simulink model "HSM_4p6U10_Motion_v01_06022022_NEW_ECC_2019a"  (R2019a)
settings: Solver=ode1  StartTime=0.0  StopTime=Inf  FixedStep=Ts  RelTol=1e-3  EnableMultiTasking=on
PostLoadFcn:
  | , if any(exist('dsrtsu_mdlpostloadfcn', 'file') == [2, 3, 6]), try dsrtsu_mdlpostloadfcn('Execute', bdroot); catch fprintf('Error in PostLoadFcn (dsrtsu_mdlpostloadfcn) for model "%s":\n %s\n', bdroot, lasterr); end, end,
values from neighbouring files (symbols this model uses):
  CDP = -1    [Parameters_4p6U10.m]
  CUP = 1    [Parameters_4p6U10.m]
  HDP = 1    [Parameters_4p6U10.m]
  HUP = -1    [Parameters_4p6U10.m]
  K1m = 1.7E-4    (= 0.00017)    [Parameters_4p6U10.m]
  K2m = 7.0E-4    (= 0.0007)    [Parameters_4p6U10.m]
  Ts = 0.0002    [Parameters_4p6U10.m]
undefined symbols (not defined in the file or in its folder): GPTRIP1SEL, GPTRIP2SEL, TZ1, TZ2
libraries: simulink_extras x25, simulink x17, c2837xDlib x11, c2802xlib x2, idelinklib_common x1
(part 2 of 3)

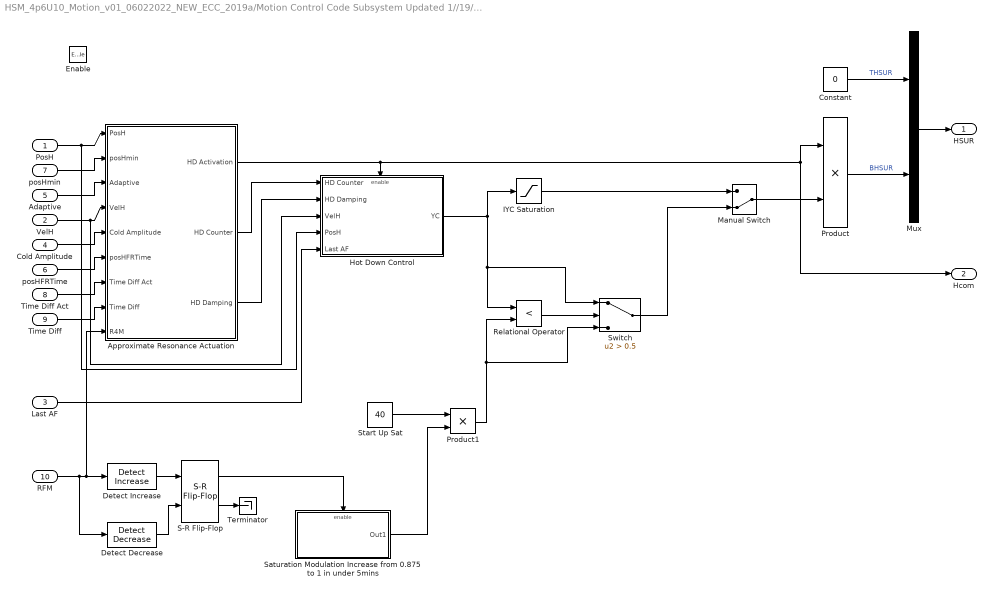
== system HSM_4p6U10_Motion_v01_06022022_NEW_ECC_2019a/Motion Control Code Subsystem Updated 1//19//21/Oscillation, Start Motion, 4 Phases Subsystem/Oscillations Subsystem Time pc No Cold Damping/Subsystem ==
  PosH : Inport
  VelH : Inport  Port=2
  Last AF : Inport  Port=3
  Cold Amplitude : Inport  Port=4
  Adaptive : Inport  Port=5
  posHFRTime : Inport  Port=6
  posHmin : Inport  Port=7
  Time Diff Act : Inport  Port=8
  Time Diff : Inport  Port=9
  RFM : Inport  Port=10
  Enable : EnablePort  StatesWhenEnabling=reset
  Approximate Resonance Actuation : Subsystem
  Constant : Constant  Value=0
  Detect Decrease : simulink/Logic and Bit Operations/Detect Decrease  vinit=0.0  OutDataTypeStr=boolean
  Detect Increase : simulink/Logic and Bit Operations/Detect Increase  vinit=0.0  OutDataTypeStr=boolean
  Hot Down Control : Subsystem  TreatAsAtomicUnit=on
  IYC Saturation : Saturate  UpperLimit=40  LowerLimit=0
  Manual Switch : ManualSwitch  CurrentSetting=0
  Mux : Mux  Inputs=2
  Product : Product
  Product1 : Product
  Relational Operator : RelationalOperator  Operator=<  OutDataTypeStr=boolean  RndMeth=Simplest
  S-R Flip-Flop : simulink_extras/Flip Flops/S-R Flip-Flop  initial_condition=0
  Saturation Modulation Increase from 0.875 to 1 in under 5mins : Subsystem
  Start Up Sat : Constant  Value=40
  Switch : Switch  Criteria=u2 > Threshold  Threshold=0.5
  Terminator : Terminator
  HSUR : Outport
  Hcom : Outport  Port=2
  wires:
  Cold Amplitude/1 -> Approximate Resonance Actuation/5(Cold Amplitude)
  PosH/1 -> Hot Down Control/4(PosH), Approximate Resonance Actuation/1(PosH)
  VelH/1 -> Hot Down Control/3(VelH), Approximate Resonance Actuation/4(VelH)
  Constant/1 -> Mux/1  "THSUR"
  Product/1 -> Mux/2  "BHSUR"
  Mux/1 -> HSUR/1
  posHmin/1 -> Approximate Resonance Actuation/2(posHmin)
  Adaptive/1 -> Approximate Resonance Actuation/3(Adaptive)
  posHFRTime/1 -> Approximate Resonance Actuation/6(posHFRTime)
  Approximate Resonance Actuation/1(HD Activation) -> Product/1, Hcom/1, Hot Down Control/Enable
  IYC Saturation/1 -> Manual Switch/1
  Approximate Resonance Actuation/2("HD Counter ") -> Hot Down Control/1(HD Counter)
  Approximate Resonance Actuation/3(HD Damping) -> Hot Down Control/2(HD Damping)
  Last AF/1 -> Hot Down Control/5(Last AF)
  Time Diff Act/1 -> Approximate Resonance Actuation/7(Time Diff Act)
  Time Diff/1 -> Approximate Resonance Actuation/8(Time Diff)
  RFM/1 -> Approximate Resonance Actuation/9(R4M), Detect Increase/1, Detect Decrease/1
  Detect Increase/1 -> S-R Flip-Flop/1
  Detect Decrease/1 -> S-R Flip-Flop/2
  S-R Flip-Flop/2 -> Terminator/1
  S-R Flip-Flop/1 -> Saturation Modulation Increase from 0.875 to 1 in under 5mins/Enable
  Saturation Modulation Increase from 0.875 to 1 in under 5mins/1(Out1) -> Product1/2
  Hot Down Control/1(YC) -> Switch/1, Relational Operator/1, IYC Saturation/1
  Manual Switch/1 -> Product/2
  Relational Operator/1 -> Switch/2
  Start Up Sat/1 -> Product1/1
  Product1/1 -> Switch/3, Relational Operator/2
  Switch/1 -> Manual Switch/2

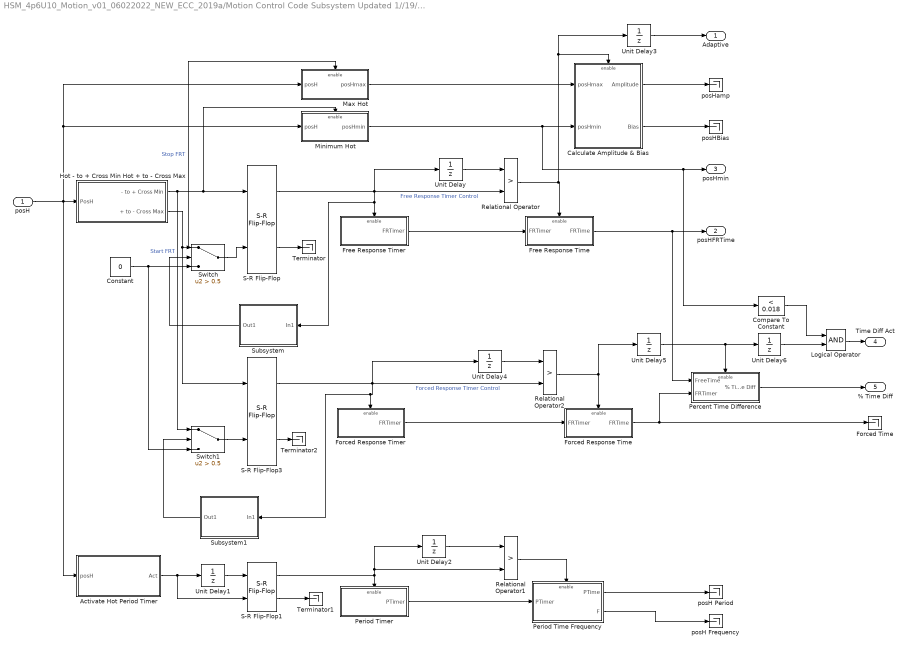
== system HSM_4p6U10_Motion_v01_06022022_NEW_ECC_2019a/Motion Control Code Subsystem Updated 1//19//21/Oscillation, Start Motion, 4 Phases Subsystem/Oscillations Subsystem Time pc No Cold Damping/System Identification & Measurement Subsystem ==
  posH : Inport
  Activate Hot Period Timer : Subsystem
  Calculate Amplitude & Bias : Subsystem
  Compare To Constant : simulink/Logic and Bit Operations/Compare To Constant  relop=<  const=0.018  OutDataTypeStr=boolean
  Constant : Constant  Value=0  OutDataTypeStr=boolean
  Forced Response Time : Subsystem
  Forced Response Timer : Subsystem
  Forced Time : Terminator
  Free Response Time : Subsystem
  Free Response Timer : Subsystem
  Hot - to + Cross Min Hot + to - Cross Max : Subsystem
  Logical Operator : Logic  AllPortsSameDT=off  OutDataTypeStr=boolean
  Max Hot : Subsystem
  Minimum Hot : Subsystem
  Percent Time Difference : Subsystem
  Period Time Frequency : Subsystem
  Period Timer : Subsystem
  Relational Operator : RelationalOperator  Operator=>  OutDataTypeStr=boolean  RndMeth=Simplest
  Relational Operator1 : RelationalOperator  Operator=>  OutDataTypeStr=boolean  RndMeth=Simplest
  Relational Operator2 : RelationalOperator  Operator=>  OutDataTypeStr=boolean  RndMeth=Simplest
  S-R Flip-Flop : simulink_extras/Flip Flops/S-R Flip-Flop  initial_condition=0
  S-R Flip-Flop1 : simulink_extras/Flip Flops/S-R Flip-Flop  initial_condition=0
  S-R Flip-Flop3 : simulink_extras/Flip Flops/S-R Flip-Flop  initial_condition=0
  Subsystem : Subsystem
  Subsystem1 : Subsystem
  Switch : Switch  Criteria=u2 > Threshold  Threshold=0.5
  Switch1 : Switch  Criteria=u2 > Threshold  Threshold=0.5
  Terminator : Terminator
  Terminator1 : Terminator
  Terminator2 : Terminator
  Unit Delay{,1..6} (7 alike) : UnitDelay  SampleTime=-1  HasFrameUpgradeWarning=on
  posH Frequency : Terminator
  posH Period : Terminator
  posHBias : Terminator
  posHamp : Terminator
  Adaptive : Outport
  posHFRTime : Outport  Port=2
  posHmin : Outport  Port=3
  Time Diff Act : Outport  Port=4
  % Time Diff : Outport  Port=5
  wires:
  Minimum Hot/1(posHmin) -> Calculate Amplitude & Bias/2(posHmin), Compare To Constant/1, posHmin/1
  S-R Flip-Flop1/1 -> Period Timer/Enable, Unit Delay2/1, Relational Operator1/2
  Period Time Frequency/1(PTime) -> posH Period/1
  S-R Flip-Flop1/2 -> Terminator1/1
  Period Time Frequency/2(F) -> posH Frequency/1
  Relational Operator1/1 -> Period Time Frequency/Enable
  Calculate Amplitude & Bias/1(Amplitude) -> posHamp/1
  Period Timer/1(PTimer) -> Period Time Frequency/1(PTimer)
  Unit Delay2/1 -> Relational Operator1/1
  Calculate Amplitude & Bias/2(Bias) -> posHBias/1
  Unit Delay1/1 -> S-R Flip-Flop1/1
  Activate Hot Period Timer/1(Act) -> Unit Delay1/1, S-R Flip-Flop1/2
  Max Hot/1(posHmax) -> Calculate Amplitude & Bias/1(posHmax)
  Free Response Timer/1(FRTimer) -> Free Response Time/1(FRTimer)
  S-R Flip-Flop/2 -> Terminator/1
  S-R Flip-Flop/1 -> Subsystem/1(In1), Free Response Timer/Enable, Relational Operator/2, Unit Delay/1  "Free Response Timer Control"
  Free Response Time/1(FRTime) -> Percent Time Difference/1(FreeTime), posHFRTime/1
  Hot - to + Cross Min Hot + to - Cross Max/1(- to + Cross Min) -> Switch1/1, S-R Flip-Flop/1, Minimum Hot/Enable  "Start FRT"
  Hot - to + Cross Min Hot + to - Cross Max/2(+ to - Cross Max) -> S-R Flip-Flop3/1, Max Hot/Enable, Switch/1  "Stop FRT"
  posH/1 -> Minimum Hot/1(posH), Max Hot/1(posH), Hot - to + Cross Min Hot + to - Cross Max/1(PosH), Activate Hot Period Timer/1(posH)
  Relational Operator/1 -> Calculate Amplitude & Bias/Enable, Unit Delay3/1, Free Response Time/Enable
  Unit Delay/1 -> Relational Operator/1
  Unit Delay3/1 -> Adaptive/1
  Switch/1 -> S-R Flip-Flop/2
  Subsystem/1(Out1) -> Switch/2
  Switch1/1 -> S-R Flip-Flop3/2
  Constant/1 -> Switch1/3, Switch/3
  Unit Delay4/1 -> Relational Operator2/1
  S-R Flip-Flop3/1 -> Subsystem1/1(In1), Forced Response Timer/Enable, Relational Operator2/2, Unit Delay4/1  "Forced Response Timer Control"
  Relational Operator2/1 -> Unit Delay5/1, Forced Response Time/Enable
  Forced Response Timer/1(FRTimer) -> Forced Response Time/1(FRTimer)
  Subsystem1/1(Out1) -> Switch1/2
  Forced Response Time/1(FRTime) -> Forced Time/1, Percent Time Difference/2(FRTimer)
  S-R Flip-Flop3/2 -> Terminator2/1
  Unit Delay5/1 -> Unit Delay6/1, Percent Time Difference/Enable
  Unit Delay6/1 -> Logical Operator/2
  Percent Time Difference/1(% Time Diff) -> % Time Diff/1
  Logical Operator/1 -> Time Diff Act/1
  Compare To Constant/1 -> Logical Operator/1

== system HSM_4p6U10_Motion_v01_06022022_NEW_ECC_2019a/Motion Control Code Subsystem Updated 1//19//21/Oscillation, Start Motion, 4 Phases Subsystem/Oscillations Subsystem Time pc No Cold Damping/Cold Resonance/Approximate Resonance Actuation ==
  PosC : Inport
  VelC : Inport  Port=2
  CD Damping : Subsystem
  CU Damping : Subsystem
  Calculate Cold Amp and Bias : Subsystem
  Subsystem1 : Subsystem
  Subsystem2 : Subsystem
  CU Activation : Outport
  CD Activation : Outport  Port=2
  CUD : Outport  Port=3
  CUCF : Outport  Port=4
  CDD : Outport  Port=5
  CDCF : Outport  Port=6
  Cold Amplitude : Outport  Port=7
  wires:
  Calculate Cold Amp and Bias/5(Cold Amplitude) -> Cold Amplitude/1
  CD Damping/1(CD Damping) -> CDD/1
  CU Damping/1(CU Damping) -> CUD/1
  Calculate Cold Amp and Bias/4(Min Cold) -> CD Damping/3(Min Cold)
  Calculate Cold Amp and Bias/1(Enable) -> CU Damping/1(Enable), CD Damping/1(Enable)
  Calculate Cold Amp and Bias/3(Max Cold) -> CU Damping/3(Max Cold)
  Calculate Cold Amp and Bias/2(Bias) -> CU Damping/2(Bias), CD Damping/2(Bias)
  PosC/1 -> CU Damping/5(posC), CD Damping/5(posC), Subsystem2/1(PosC), Calculate Cold Amp and Bias/1(posC)
  Subsystem1/1(Top Safety Limit) -> Subsystem2/3(Top Safety Limit), CU Damping/4(TSL), Calculate Cold Amp and Bias/5(TSL)
  Subsystem1/2(Bottom Safety Limit) -> CD Damping/4(BSL), Subsystem2/4(Bot Safety Limit), Calculate Cold Amp and Bias/6(BSL)
  VelC/1 -> Subsystem2/2(VelC), Calculate Cold Amp and Bias/2(velC)
  Subsystem2/1(CU Activation) -> CU Activation/1, Calculate Cold Amp and Bias/3(CU Deact)
  Subsystem2/2(CD Activation) -> CD Activation/1, Calculate Cold Amp and Bias/4(CD Deact)
  CU Damping/2(CU Constant Force) -> CUCF/1
  CD Damping/2(CD Constant Force) -> CDCF/1

== system HSM_4p6U10_Motion_v01_06022022_NEW_ECC_2019a/Motion Control Code Subsystem Updated 1//19//21/Oscillation, Start Motion, 4 Phases Subsystem/Oscillations Subsystem Time pc No Cold Damping/Cold Resonance/Cold Down Control ==
  VelC : Inport
  PosC : Inport  Port=2
  CDD : Inport  Port=3
  CDCF : Inport  Port=4
  Enable : EnablePort  StatesWhenEnabling=reset
  Damping Coefficient : Constant  Value=100
  Gain : Gain
  Gain1 : Gain  Gain=0
  Product : Product
  Sum : Sum  Inputs=|++
  Terminator : Terminator
  Unity Gain Scaling : Subsystem
  IBC : Outport
  wires:
  Gain1/1 -> Product/2
  PosC/1 -> Unity Gain Scaling/2(x)
  Unity Gain Scaling/1(i) -> IBC/1
  VelC/1 -> Product/1
  Sum/1 -> Unity Gain Scaling/1(u)  "Negative Damping"
  Damping Coefficient/1 -> Terminator/1
  Product/1 -> Sum/1  "Negative Damping"
  CDCF/1 -> Gain/1
  Gain/1 -> Sum/2
  CDD/1 -> Gain1/1

== system HSM_4p6U10_Motion_v01_06022022_NEW_ECC_2019a/Motion Control Code Subsystem Updated 1//19//21/Oscillation, Start Motion, 4 Phases Subsystem/Oscillations Subsystem Time pc No Cold Damping/Cold Resonance/Cold Up Control ==
  VelC : Inport
  PosC : Inport  Port=2
  CUD : Inport  Port=3
  CUCF : Inport  Port=4
  Enable : EnablePort  StatesWhenEnabling=reset
  Acceleration to Current : Subsystem
  Damping Coefficient : Constant  Value=250
  Gain : Gain
  Gain1 : Gain  Gain=0
  Product : Product
  Sum : Sum  Inputs=|++
  Terminator : Terminator
  IRC : Outport
  wires:
  CUD/1 -> Gain1/1
  VelC/1 -> Product/1
  PosC/1 -> Acceleration to Current/2(X)
  Sum/1 -> Acceleration to Current/1(U)
  Acceleration to Current/1(I) -> IRC/1
  Damping Coefficient/1 -> Terminator/1
  Product/1 -> Sum/1
  CUCF/1 -> Gain/1
  Gain/1 -> Sum/2
  Gain1/1 -> Product/2

== system HSM_4p6U10_Motion_v01_06022022_NEW_ECC_2019a/Motion Control Code Subsystem Updated 1//19//21/Oscillation, Start Motion, 4 Phases Subsystem/Oscillations Subsystem Time pc No Cold Damping/Initial Applied Force/Grab and Hold Last Applied Force ==
  AF : Inport
  Enable : EnablePort  StatesWhenEnabling=reset
  Last AF : Outport
  wires:
  AF/1 -> Last AF/1

== system HSM_4p6U10_Motion_v01_06022022_NEW_ECC_2019a/Motion Control Code Subsystem Updated 1//19//21/Oscillation, Start Motion, 4 Phases Subsystem/Oscillations Subsystem Time pc No Cold Damping/Initial Applied Force/Unity Gain Scaling ==
  u : Inport
  x : Inport  Port=2
  Constant6 : Constant  Value=K2m
  Gain1 : Gain  Gain=-1/K1m
  IYC^2 Saturation : Saturate  UpperLimit=3600  LowerLimit=0
  Math Function4 : Math  Operator=square  SaturateOnIntegerOverflow=on
  Product1 : Product
  Sqrt : Sqrt  SaturateOnIntegerOverflow=on
  Sum3 : Sum
  i : Outport
  wires:
  u/1 -> Gain1/1
  Sum3/1 -> Math Function4/1
  Constant6/1 -> Sum3/1
  Math Function4/1 -> Product1/2
  x/1 -> Sum3/2
  Gain1/1 -> Product1/1
  Product1/1 -> IYC^2 Saturation/1
  Sqrt/1 -> i/1
  IYC^2 Saturation/1 -> Sqrt/1

== system HSM_4p6U10_Motion_v01_06022022_NEW_ECC_2019a/Motion Control Code Subsystem Updated 1//19//21/Oscillation, Start Motion, 4 Phases Subsystem/Oscillations Subsystem Time pc No Cold Damping/Subsystem/Approximate Resonance Actuation ==
  PosH : Inport
  posHmin : Inport  Port=2
  Adaptive : Inport  Port=3
  VelH : Inport  Port=4
  Cold Amplitude : Inport  Port=5
  posHFRTime : Inport  Port=6
  Time Diff Act : Inport  Port=7
  Time Diff : Inport  Port=8
  R4M : Inport  Port=9
  Subsystem : Subsystem
  Subsystem1 : Subsystem
  Subsystem2 : Subsystem
  HD Activation : Outport
  "HD Counter " : Outport  Port=2
  HD Damping : Outport  Port=3
  wires:
  posHFRTime/1 -> Subsystem2/4(posHFRTime)
  Cold Amplitude/1 -> Subsystem1/1(Cold Amplitude)
  VelH/1 -> Subsystem2/2(VelH)
  Subsystem1/1(Bottom Safety Limit) -> Subsystem/3(BSL), Subsystem2/3(Bot Safety Limit)
  PosH/1 -> Subsystem2/1(PosH)
  Subsystem2/1(HD Activation) -> HD Activation/1
  posHmin/1 -> Subsystem/1(posHmin)
  Adaptive/1 -> Subsystem/2(Adaptive)
  Subsystem/1("HD Counter ") -> "HD Counter "/1
  Subsystem/2(HD Damping) -> HD Damping/1
  Time Diff Act/1 -> Subsystem/4(Time Diff Act)
  Time Diff/1 -> Subsystem/5(Time Diff)
  R4M/1 -> Subsystem1/2(R4M)

== system HSM_4p6U10_Motion_v01_06022022_NEW_ECC_2019a/Motion Control Code Subsystem Updated 1//19//21/Oscillation, Start Motion, 4 Phases Subsystem/Oscillations Subsystem Time pc No Cold Damping/Subsystem/Hot Down Control ==
  HD Counter : Inport
  HD Damping : Inport  Port=2
  VelH : Inport  Port=3
  PosH : Inport  Port=4
  Last AF : Inport  Port=5
  Enable : EnablePort  StatesWhenEnabling=reset
  FF_Hot_Down : Constant  Value=-50
  Gain1 : Gain
  Last AF Multiplier : Gain  Gain=0.3
  Product : Product
  Saturation1 : Saturate  UpperLimit=200  LowerLimit=-10000
  Sum : Sum  Inputs=+++
  Sum1 : Sum  Inputs=|++
  Unity Gain Scaling : Subsystem
  YC : Outport
  wires:
  Unity Gain Scaling/1(i) -> YC/1
  Sum/1 -> Unity Gain Scaling/1(u)  "Net Force"
  PosH/1 -> Unity Gain Scaling/2(x)
  HD Damping/1 -> Product/2
  Last AF Multiplier/1 -> Sum1/1
  HD Counter/1 -> Gain1/1
  Saturation1/1 -> Sum/3
  Sum1/1 -> Saturation1/1  "Offset Force"
  Gain1/1 -> Sum1/2
  Product/1 -> Sum/2  "Negative Damping"
  Last AF/1 -> Last AF Multiplier/1
  VelH/1 -> Product/1
  FF_Hot_Down/1 -> Sum/1  "Coloumb Friction Compensation"

== system HSM_4p6U10_Motion_v01_06022022_NEW_ECC_2019a/Motion Control Code Subsystem Updated 1//19//21/Oscillation, Start Motion, 4 Phases Subsystem/Oscillations Subsystem Time pc No Cold Damping/Subsystem/Saturation Modulation Increase from 0.875 to 1 in under 5mins ==
  Enable : EnablePort  StatesWhenEnabling=reset
  Constant : Constant
  Gain : Gain  Gain=0.001
  Integrator : Integrator  LimitOutput=on  UpperSaturationLimit=300  LowerSaturationLimit=0
  Limit Saturation : Saturate  UpperLimit=1  LowerLimit=0.875
  Sum : Sum  Inputs=|++
  Unit : Constant  Value=0.875
  Out1 : Outport
  wires:
  Limit Saturation/1 -> Out1/1
  Sum/1 -> Limit Saturation/1
  Unit/1 -> Sum/2
  Gain/1 -> Sum/1
  Integrator/1 -> Gain/1
  Constant/1 -> Integrator/1

== system HSM_4p6U10_Motion_v01_06022022_NEW_ECC_2019a/Motion Control Code Subsystem Updated 1//19//21/Oscillation, Start Motion, 4 Phases Subsystem/Oscillations Subsystem Time pc No Cold Damping/System Identification & Measurement Subsystem/Activate Hot Period Timer ==
  posH : Inport
  Constant : Constant  Value=0.025
  Logical Operator : Logic  AllPortsSameDT=off  OutDataTypeStr=boolean
  Relational Operator1 : RelationalOperator  Operator=<  OutDataTypeStr=boolean  RndMeth=Simplest
  Relational Operator2 : RelationalOperator  OutDataTypeStr=boolean  RndMeth=Simplest
  Unit Delay1 : UnitDelay  SampleTime=-1  HasFrameUpgradeWarning=on
  Act : Outport
  wires:
  Relational Operator2/1 -> Logical Operator/2
  Constant/1 -> Relational Operator1/2, Relational Operator2/2
  Unit Delay1/1 -> Relational Operator1/1
  Relational Operator1/1 -> Logical Operator/1
  Logical Operator/1 -> Act/1
  posH/1 -> Relational Operator2/1, Unit Delay1/1

== system HSM_4p6U10_Motion_v01_06022022_NEW_ECC_2019a/Motion Control Code Subsystem Updated 1//19//21/Oscillation, Start Motion, 4 Phases Subsystem/Oscillations Subsystem Time pc No Cold Damping/System Identification & Measurement Subsystem/Calculate Amplitude & Bias ==
  posHmax : Inport
  posHmin : Inport  Port=2
  Enable : EnablePort  StatesWhenEnabling=reset
  Gain : Gain  Gain=1/2
  Sum : Sum
  Sum1 : Sum  Inputs=+-
  Amplitude : Outport
  Bias : Outport  Port=2
  wires:
  Sum1/1 -> Amplitude/1
  Gain/1 -> Sum1/2, Bias/1
  Sum/1 -> Gain/1
  posHmin/1 -> Sum/2
  posHmax/1 -> Sum/1, Sum1/1

== system HSM_4p6U10_Motion_v01_06022022_NEW_ECC_2019a/Motion Control Code Subsystem Updated 1//19//21/Oscillation, Start Motion, 4 Phases Subsystem/Oscillations Subsystem Time pc No Cold Damping/System Identification & Measurement Subsystem/Forced Response Time ==
  FRTimer : Inport
  Enable : EnablePort  StatesWhenEnabling=reset
  FRTime : Outport
  wires:
  FRTimer/1 -> FRTime/1

== system HSM_4p6U10_Motion_v01_06022022_NEW_ECC_2019a/Motion Control Code Subsystem Updated 1//19//21/Oscillation, Start Motion, 4 Phases Subsystem/Oscillations Subsystem Time pc No Cold Damping/System Identification & Measurement Subsystem/Forced Response Timer ==
  Enable : EnablePort  StatesWhenEnabling=reset
  Constant : Constant
  Integrator : Integrator
  FRTimer : Outport
  wires:
  Constant/1 -> Integrator/1
  Integrator/1 -> FRTimer/1

== system HSM_4p6U10_Motion_v01_06022022_NEW_ECC_2019a/Motion Control Code Subsystem Updated 1//19//21/Oscillation, Start Motion, 4 Phases Subsystem/Oscillations Subsystem Time pc No Cold Damping/System Identification & Measurement Subsystem/Free Response Time ==
  FRTimer : Inport
  Enable : EnablePort  StatesWhenEnabling=reset
  FRTime : Outport
  wires:
  FRTimer/1 -> FRTime/1

== system HSM_4p6U10_Motion_v01_06022022_NEW_ECC_2019a/Motion Control Code Subsystem Updated 1//19//21/Oscillation, Start Motion, 4 Phases Subsystem/Oscillations Subsystem Time pc No Cold Damping/System Identification & Measurement Subsystem/Free Response Timer ==
  Enable : EnablePort  StatesWhenEnabling=reset
  Constant : Constant
  Integrator : Integrator
  FRTimer : Outport
  wires:
  Constant/1 -> Integrator/1
  Integrator/1 -> FRTimer/1

== system HSM_4p6U10_Motion_v01_06022022_NEW_ECC_2019a/Motion Control Code Subsystem Updated 1//19//21/Oscillation, Start Motion, 4 Phases Subsystem/Oscillations Subsystem Time pc No Cold Damping/System Identification & Measurement Subsystem/Hot - to + Cross Min Hot + to - Cross Max ==
  PosH : Inport
  Delay : Delay  DelayLength=12
  Delay1 : Delay  DelayLength=12
  Logical Operator1 : Logic  AllPortsSameDT=off  OutDataTypeStr=boolean
  Logical Operator2 : Logic  AllPortsSameDT=off  OutDataTypeStr=boolean
  Relational Operator1 : RelationalOperator  Operator=<  OutDataTypeStr=boolean  RndMeth=Simplest
  Relational Operator2 : RelationalOperator  Operator=>  OutDataTypeStr=boolean  RndMeth=Simplest
  Relational Operator3 : RelationalOperator  Operator=>  OutDataTypeStr=boolean  RndMeth=Simplest
  Relational Operator4 : RelationalOperator  Operator=<  OutDataTypeStr=boolean  RndMeth=Simplest
  - to + Cross Min : Outport
  + to - Cross Max : Outport  Port=2
  wires:
  PosH/1 -> Relational Operator1/1, Delay/1, Relational Operator3/1
  Relational Operator4/1 -> Logical Operator1/2
  Relational Operator3/1 -> Logical Operator1/1
  Delay/1 -> Relational Operator3/2, Relational Operator4/1, Relational Operator2/1, Relational Operator1/2, Delay1/1
  Logical Operator1/1 -> - to + Cross Min/1
  Delay1/1 -> Relational Operator4/2, Relational Operator2/2
  Logical Operator2/1 -> + to - Cross Max/1
  Relational Operator2/1 -> Logical Operator2/2
  Relational Operator1/1 -> Logical Operator2/1

== system HSM_4p6U10_Motion_v01_06022022_NEW_ECC_2019a/Motion Control Code Subsystem Updated 1//19//21/Oscillation, Start Motion, 4 Phases Subsystem/Oscillations Subsystem Time pc No Cold Damping/System Identification & Measurement Subsystem/Max Hot ==
  posH : Inport
  Enable : EnablePort  StatesWhenEnabling=reset
  posHmax : Outport
  wires:
  posH/1 -> posHmax/1

== system HSM_4p6U10_Motion_v01_06022022_NEW_ECC_2019a/Motion Control Code Subsystem Updated 1//19//21/Oscillation, Start Motion, 4 Phases Subsystem/Oscillations Subsystem Time pc No Cold Damping/System Identification & Measurement Subsystem/Minimum Hot ==
  posH : Inport
  Enable : EnablePort  StatesWhenEnabling=reset
  posHmin : Outport
  wires:
  posH/1 -> posHmin/1

== system HSM_4p6U10_Motion_v01_06022022_NEW_ECC_2019a/Motion Control Code Subsystem Updated 1//19//21/Oscillation, Start Motion, 4 Phases Subsystem/Oscillations Subsystem Time pc No Cold Damping/System Identification & Measurement Subsystem/Percent Time Difference ==
  FreeTime : Inport
  FRTimer : Inport  Port=2
  Enable : EnablePort  StatesWhenEnabling=reset
  Divide : Product  Inputs=*/
  Gain : Gain  Gain=100
  Sum : Sum  Inputs=+-
  % Time Diff : Outport
  wires:
  FRTimer/1 -> Sum/2
  FreeTime/1 -> Divide/2, Sum/1
  Sum/1 -> Divide/1
  Divide/1 -> Gain/1
  Gain/1 -> % Time Diff/1

== system HSM_4p6U10_Motion_v01_06022022_NEW_ECC_2019a/Motion Control Code Subsystem Updated 1//19//21/Oscillation, Start Motion, 4 Phases Subsystem/Oscillations Subsystem Time pc No Cold Damping/System Identification & Measurement Subsystem/Period Time Frequency ==
  PTimer : Inport
  Enable : EnablePort  StatesWhenEnabling=reset
  Math Function : Math  Operator=reciprocal  SaturateOnIntegerOverflow=on
  PTime : Outport
  F : Outport  Port=2
  wires:
  Math Function/1 -> F/1
  PTimer/1 -> PTime/1, Math Function/1

== system HSM_4p6U10_Motion_v01_06022022_NEW_ECC_2019a/Motion Control Code Subsystem Updated 1//19//21/Oscillation, Start Motion, 4 Phases Subsystem/Oscillations Subsystem Time pc No Cold Damping/System Identification & Measurement Subsystem/Period Timer ==
  Enable : EnablePort  StatesWhenEnabling=reset
  Constant : Constant
  Integrator : Integrator
  PTimer : Outport
  wires:
  Integrator/1 -> PTimer/1
  Constant/1 -> Integrator/1

== system HSM_4p6U10_Motion_v01_06022022_NEW_ECC_2019a/Motion Control Code Subsystem Updated 1//19//21/Oscillation, Start Motion, 4 Phases Subsystem/Oscillations Subsystem Time pc No Cold Damping/System Identification & Measurement Subsystem/Subsystem ==
  In1 : Inport
  Compare To Constant : simulink/Logic and Bit Operations/Compare To Constant  relop=>  const=0.01  OutDataTypeStr=boolean
  Data Type Conversion : DataTypeConversion  OutDataTypeStr=double
  Integrator : Integrator  ExternalReset=rising
  Logical Operator : Logic  Operator=NOT  AllPortsSameDT=off  OutDataTypeStr=boolean
  Unit Delay4 : UnitDelay  SampleTime=-1  HasFrameUpgradeWarning=on
  Out1 : Outport
  wires:
  In1/1 -> Data Type Conversion/1
  Data Type Conversion/1 -> Logical Operator/1, Integrator/1
  Unit Delay4/1 -> Integrator/2
  Compare To Constant/1 -> Out1/1
  Integrator/1 -> Compare To Constant/1
  Logical Operator/1 -> Unit Delay4/1

== system HSM_4p6U10_Motion_v01_06022022_NEW_ECC_2019a/Motion Control Code Subsystem Updated 1//19//21/Oscillation, Start Motion, 4 Phases Subsystem/Oscillations Subsystem Time pc No Cold Damping/System Identification & Measurement Subsystem/Subsystem1 ==
  In1 : Inport
  Compare To Constant : simulink/Logic and Bit Operations/Compare To Constant  relop=>  const=0.01  OutDataTypeStr=boolean
  Data Type Conversion : DataTypeConversion  OutDataTypeStr=double
  Integrator : Integrator  ExternalReset=rising
  Logical Operator : Logic  Operator=NOT  AllPortsSameDT=off  OutDataTypeStr=boolean
  Unit Delay4 : UnitDelay  SampleTime=-1  HasFrameUpgradeWarning=on
  Out1 : Outport
  wires:
  Logical Operator/1 -> Unit Delay4/1
  Integrator/1 -> Compare To Constant/1
  Compare To Constant/1 -> Out1/1
  Unit Delay4/1 -> Integrator/2
  Data Type Conversion/1 -> Integrator/1, Logical Operator/1
  In1/1 -> Data Type Conversion/1

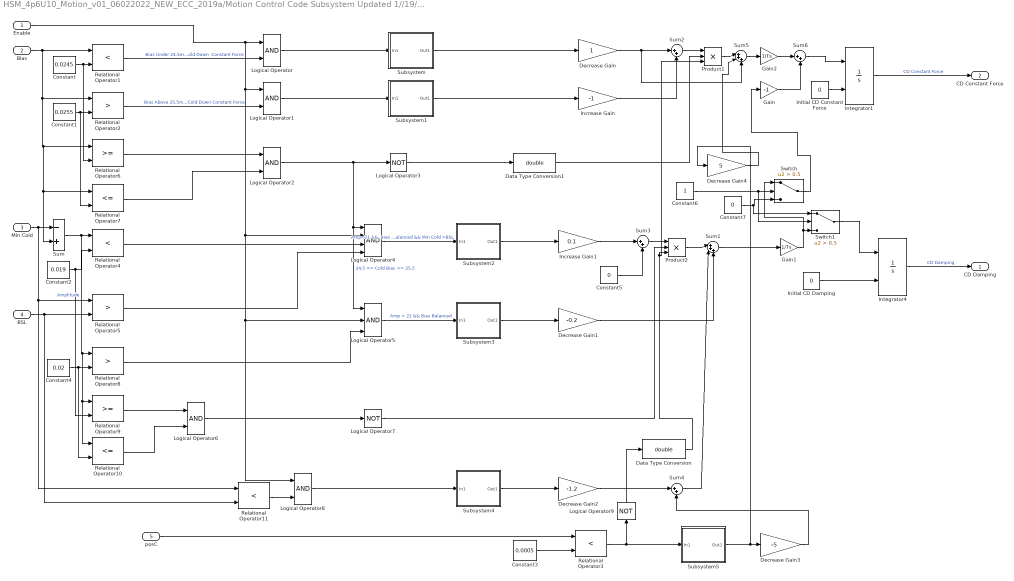
== system HSM_4p6U10_Motion_v01_06022022_NEW_ECC_2019a/Motion Control Code Subsystem Updated 1//19//21/Oscillation, Start Motion, 4 Phases Subsystem/Oscillations Subsystem Time pc No Cold Damping/Cold Resonance/Approximate Resonance Actuation/CD Damping ==
  Enable : Inport
  Bias : Inport  Port=2
  Min Cold : Inport  Port=3
  BSL : Inport  Port=4
  posC : Inport  Port=5
  Constant : Constant  Value=0.0245
  Constant1 : Constant  Value=0.0255
  Constant2 : Constant  Value=0.019
  Constant3 : Constant  Value=0.0005
  Constant4 : Constant  Value=0.02
  Constant5 : Constant  Value=0
  Constant6 : Constant
  Constant7 : Constant  Value=0
  Data Type Conversion : DataTypeConversion  OutDataTypeStr=double
  Data Type Conversion1 : DataTypeConversion  OutDataTypeStr=double
  Decrease Gain : Gain  OutDataTypeStr=double
  Decrease Gain1 : Gain  Gain=-0.2  OutDataTypeStr=double
  Decrease Gain2 : Gain  Gain=-1.2  OutDataTypeStr=double
  Decrease Gain3 : Gain  Gain=-5  OutDataTypeStr=double
  Decrease Gain4 : Gain  Gain=5  OutDataTypeStr=double
  Gain : Gain  Gain=-1
  Gain1 : Gain  Gain=1/Ts
  Gain2 : Gain  Gain=1/Ts
  Increase Gain : Gain  Gain=-1  OutDataTypeStr=double
  Increase Gain1 : Gain  Gain=0.1  OutDataTypeStr=double
  Initial CD Constant Force : Constant  Value=0  OutDataTypeStr=double
  Initial CD Damping : Constant  Value=0  OutDataTypeStr=double
  Integrator1 : Integrator  InitialConditionSource=external  LimitOutput=on  UpperSaturationLimit=200  LowerSaturationLimit=-2000
  Integrator4 : Integrator  InitialConditionSource=external  LimitOutput=on  UpperSaturationLimit=2000  LowerSaturationLimit=0
  Logical Operator{,1..2,6,8} (5 alike) : Logic  AllPortsSameDT=off  OutDataTypeStr=boolean
  Logical Operator3 : Logic  Operator=NOT  AllPortsSameDT=off  OutDataTypeStr=boolean
  Logical Operator4 : Logic  Inputs=4  AllPortsSameDT=off  OutDataTypeStr=boolean
  Logical Operator5 : Logic  Inputs=3  AllPortsSameDT=off  OutDataTypeStr=boolean
  Logical Operator7 : Logic  Operator=NOT  AllPortsSameDT=off  OutDataTypeStr=boolean
  Logical Operator9 : Logic  Operator=NOT  AllPortsSameDT=off  OutDataTypeStr=boolean
  Product1 : Product  Inputs=3
  Product2 : Product  Inputs=3
  Relational Operator{1,3..4,11} (4 alike) : RelationalOperator  Operator=<  OutDataTypeStr=boolean  RndMeth=Simplest
  Relational Operator10 : RelationalOperator  Operator=<=  OutDataTypeStr=boolean  RndMeth=Simplest
  Relational Operator2 : RelationalOperator  Operator=>  OutDataTypeStr=boolean  RndMeth=Simplest
  Relational Operator5 : RelationalOperator  Operator=>  OutDataTypeStr=boolean  RndMeth=Simplest
  Relational Operator6 : RelationalOperator  OutDataTypeStr=boolean  RndMeth=Simplest
  Relational Operator7 : RelationalOperator  Operator=<=  OutDataTypeStr=boolean  RndMeth=Simplest
  Relational Operator8 : RelationalOperator  Operator=>  OutDataTypeStr=boolean  RndMeth=Simplest
  Relational Operator9 : RelationalOperator  OutDataTypeStr=boolean  RndMeth=Simplest
  Subsystem : Subsystem
  Subsystem1 : Subsystem
  Subsystem2 : Subsystem
  Subsystem3 : Subsystem
  Subsystem4 : Subsystem
  Subsystem5 : Subsystem
  Sum : Sum  Inputs=-+
  Sum1 : Sum  Inputs=|+++
  Sum{2..4,6} (4 alike) : Sum  Inputs=|++
  Sum5 : Sum  Inputs=|+++
  Switch : Switch  Criteria=u2 > Threshold  Threshold=0.5
  Switch1 : Switch  Criteria=u2 > Threshold  Threshold=0.5
  CD Damping : Outport
  CD Constant Force : Outport  Port=2
  wires:
  Sum6/1 -> Integrator1/1
  Gain/1 -> Sum6/2
  Gain1/1 -> Switch1/3, Switch/1
  Constant6/1 -> Switch/2, Switch1/2
  Switch1/1 -> Integrator4/1
  Sum1/1 -> Gain1/1
  Constant7/1 -> Switch/3, Switch1/1
  Switch/1 -> Gain/1
  Logical Operator9/1 -> Data Type Conversion/1
  Data Type Conversion1/1 -> Product1/2
  Constant5/1 -> Sum3/2
  Decrease Gain4/1 -> Sum5/2
  Product1/1 -> Sum5/1
  Data Type Conversion/1 -> Product2/3, Product1/3
  Decrease Gain3/1 -> Sum4/2
  Decrease Gain2/1 -> Sum4/1
  Subsystem5/1(Out1) -> Decrease Gain3/1, Decrease Gain4/1
  Initial CD Damping/1 -> Integrator4/2
  Sum4/1 -> Sum1/2
  Subsystem4/1(Out1) -> Decrease Gain2/1
  Logical Operator8/1 -> Subsystem4/1(In1)
  Relational Operator11/1 -> Logical Operator8/2
  Logical Operator7/1 -> Product2/2
  Logical Operator6/1 -> Logical Operator7/1
  Relational Operator10/1 -> Logical Operator6/2
  Relational Operator9/1 -> Logical Operator6/1
  Sum3/1 -> Product2/1
  Decrease Gain1/1 -> Sum1/3
  Increase Gain1/1 -> Sum3/1
  Subsystem3/1(Out1) -> Decrease Gain1/1
  Logical Operator5/1 -> Subsystem3/1(In1)  "Amp > 22 && Bias Balanced"
  Relational Operator8/1 -> Logical Operator5/3
  Constant4/1 -> Relational Operator8/2, Relational Operator10/2
  Subsystem2/1(Out1) -> Increase Gain1/1
  Relational Operator5/1 -> Logical Operator4/4
  Relational Operator4/1 -> Logical Operator4/3
  Logical Operator4/1 -> Subsystem2/1(In1)  "Amp<21 &&  Bias Balanced && Min Cold >BSL"
  Constant2/1 -> Relational Operator4/2, Relational Operator9/2
  Sum/1 -> Relational Operator8/1, Relational Operator9/1, Relational Operator10/1, Relational Operator4/1  "Amplitude"
  Logical Operator3/1 -> Data Type Conversion1/1
  Sum2/1 -> Product1/1
  Logical Operator2/1 -> Logical Operator3/1, Logical Operator4/1, Logical Operator5/1  "24.5 <= Cold Bias <= 25.5"
  Subsystem1/1(Out1) -> Increase Gain/1
  Logical Operator1/1 -> Subsystem1/1(In1)
  Subsystem/1(Out1) -> Decrease Gain/1
  Logical Operator/1 -> Subsystem/1(In1)
  Relational Operator7/1 -> Logical Operator2/2
  Relational Operator6/1 -> Logical Operator2/1
  Constant/1 -> Relational Operator1/2, Relational Operator6/2
  Bias/1 -> Relational Operator1/1, Relational Operator2/1, Relational Operator6/1, Sum/2, Relational Operator7/1
  Relational Operator2/1 -> Logical Operator1/2  "Bias Above 25.5mm Decrease Cold Down Constant Force"
  Constant1/1 -> Relational Operator2/2, Relational Operator7/2
  Enable/1 -> Logical Operator/1, Logical Operator1/1, Logical Operator4/2, Logical Operator5/2, Logical Operator8/1
  Relational Operator1/1 -> Logical Operator/2  "Bias Under 24.5mm  Decrease Cold Down  Constant Force"
  Min Cold/1 -> Sum/1, Relational Operator5/1, Relational Operator11/1
  posC/1 -> Relational Operator3/1
  BSL/1 -> Relational Operator5/2, Relational Operator11/2
  Integrator4/1 -> CD Damping/1  "CD Damping"
  Constant3/1 -> Relational Operator3/2
  Product2/1 -> Sum1/1
  Initial CD Constant Force/1 -> Integrator1/2
  Integrator1/1 -> CD Constant Force/1  "CD Constant Force"
  Relational Operator3/1 -> Logical Operator9/1, Subsystem5/1(In1)
  Gain2/1 -> Sum6/1
  Sum5/1 -> Gain2/1
  Decrease Gain/1 -> Sum2/1, Sum5/3
  Increase Gain/1 -> Sum2/2

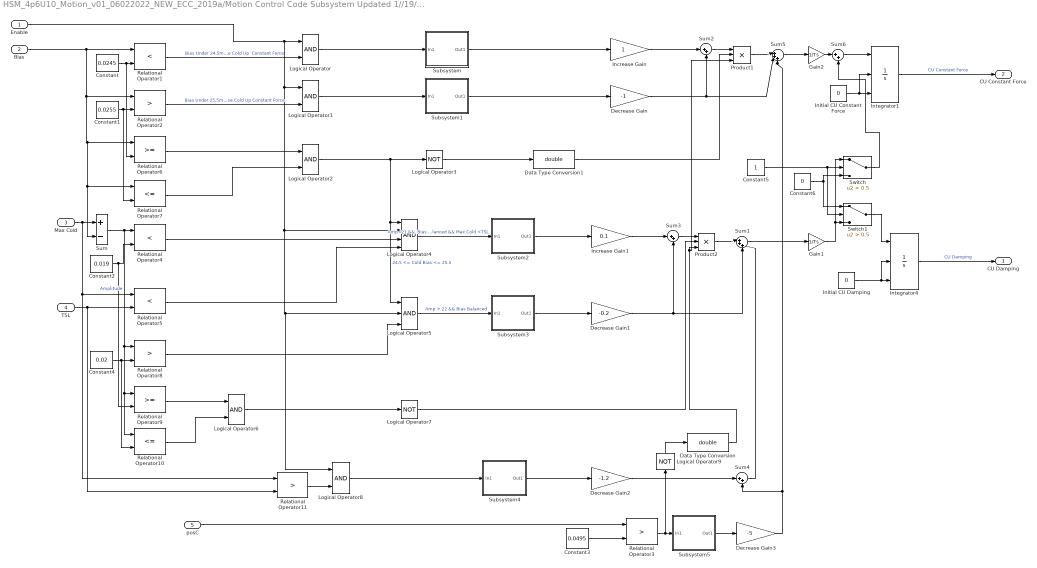
== system HSM_4p6U10_Motion_v01_06022022_NEW_ECC_2019a/Motion Control Code Subsystem Updated 1//19//21/Oscillation, Start Motion, 4 Phases Subsystem/Oscillations Subsystem Time pc No Cold Damping/Cold Resonance/Approximate Resonance Actuation/CU Damping ==
  Enable : Inport
  Bias : Inport  Port=2
  Max Cold : Inport  Port=3
  TSL : Inport  Port=4
  posC : Inport  Port=5
  Constant : Constant  Value=0.0245
  Constant1 : Constant  Value=0.0255
  Constant2 : Constant  Value=0.019
  Constant3 : Constant  Value=0.0495
  Constant4 : Constant  Value=0.02
  Constant5 : Constant
  Constant6 : Constant  Value=0
  Data Type Conversion : DataTypeConversion  OutDataTypeStr=double
  Data Type Conversion1 : DataTypeConversion  OutDataTypeStr=double
  Decrease Gain : Gain  Gain=-1  OutDataTypeStr=double
  Decrease Gain1 : Gain  Gain=-0.2  OutDataTypeStr=double
  Decrease Gain2 : Gain  Gain=-1.2  OutDataTypeStr=double
  Decrease Gain3 : Gain  Gain=-5  OutDataTypeStr=double
  Gain1 : Gain  Gain=1/Ts
  Gain2 : Gain  Gain=1/Ts
  Increase Gain : Gain  OutDataTypeStr=double
  Increase Gain1 : Gain  Gain=0.1  OutDataTypeStr=double
  Initial CU Constant Force : Constant  Value=0  OutDataTypeStr=double
  Initial CU Damping : Constant  Value=0  OutDataTypeStr=double
  Integrator1 : Integrator  ExternalReset=rising  InitialConditionSource=external  LimitOutput=on  UpperSaturationLimit=2000  LowerSaturationLimit=0
  Integrator4 : Integrator  ExternalReset=falling  InitialConditionSource=external  LimitOutput=on  UpperSaturationLimit=2000  LowerSaturationLimit=0
  Logical Operator{,1..2,6,8} (5 alike) : Logic  AllPortsSameDT=off  OutDataTypeStr=boolean
  Logical Operator3 : Logic  Operator=NOT  AllPortsSameDT=off  OutDataTypeStr=boolean
  Logical Operator4 : Logic  Inputs=4  AllPortsSameDT=off  OutDataTypeStr=boolean
  Logical Operator5 : Logic  Inputs=3  AllPortsSameDT=off  OutDataTypeStr=boolean
  Logical Operator7 : Logic  Operator=NOT  AllPortsSameDT=off  OutDataTypeStr=boolean
  Logical Operator9 : Logic  Operator=NOT  AllPortsSameDT=off  OutDataTypeStr=boolean
  Product1 : Product  Inputs=3
  Product2 : Product  Inputs=3
  Relational Operator1 : RelationalOperator  Operator=<  OutDataTypeStr=boolean  RndMeth=Simplest
  Relational Operator10 : RelationalOperator  Operator=<=  OutDataTypeStr=boolean  RndMeth=Simplest
  Relational Operator{2..3,8,11} (4 alike) : RelationalOperator  Operator=>  OutDataTypeStr=boolean  RndMeth=Simplest
  Relational Operator4 : RelationalOperator  Operator=<  OutDataTypeStr=boolean  RndMeth=Simplest
  Relational Operator5 : RelationalOperator  Operator=<  OutDataTypeStr=boolean  RndMeth=Simplest
  Relational Operator6 : RelationalOperator  OutDataTypeStr=boolean  RndMeth=Simplest
  Relational Operator7 : RelationalOperator  Operator=<=  OutDataTypeStr=boolean  RndMeth=Simplest
  Relational Operator9 : RelationalOperator  OutDataTypeStr=boolean  RndMeth=Simplest
  Subsystem : Subsystem
  Subsystem1 : Subsystem
  Subsystem2 : Subsystem
  Subsystem3 : Subsystem
  Subsystem4 : Subsystem
  Subsystem5 : Subsystem
  Sum : Sum  Inputs=+-
  Sum1 : Sum  Inputs=|+++
  Sum{2..4,6} (4 alike) : Sum  Inputs=|++
  Sum5 : Sum  Inputs=|+++
  Switch : Switch  Criteria=u2 > Threshold  Threshold=0.5
  Switch1 : Switch  Criteria=u2 > Threshold  Threshold=0.5
  CU Damping : Outport
  CU Constant Force : Outport  Port=2
  wires:
  Switch1/1 -> Integrator4/1
  Switch/1 -> Sum6/2
  Gain2/1 -> Sum6/1
  Constant6/1 -> Switch/3, Switch1/1
  Constant5/1 -> Switch/2, Switch1/2
  Product1/1 -> Sum5/1
  Data Type Conversion1/1 -> Product1/2
  Logical Operator9/1 -> Data Type Conversion/1
  Data Type Conversion/1 -> Product2/3, Product1/3
  Decrease Gain3/1 -> Sum5/3, Sum4/2
  Decrease Gain2/1 -> Sum4/1
  Subsystem5/1(Out1) -> Decrease Gain3/1
  Relational Operator3/1 -> Subsystem5/1(In1), Logical Operator9/1
  Decrease Gain/1 -> Sum2/2, Sum5/2
  Increase Gain/1 -> Sum2/1
  Sum5/1 -> Gain2/1
  Sum6/1 -> Integrator1/1
  Integrator1/1 -> CU Constant Force/1  "CU Constant Force"
  Initial CU Constant Force/1 -> Integrator1/3, Integrator1/2
  Sum1/1 -> Gain1/1
  Product2/1 -> Sum1/1
  Constant3/1 -> Relational Operator3/2
  Initial CU Damping/1 -> Integrator4/3, Integrator4/2
  Integrator4/1 -> CU Damping/1  "CU Damping"
  Gain1/1 -> Switch/1, Switch1/3
  TSL/1 -> Relational Operator11/2, Relational Operator5/2
  posC/1 -> Relational Operator3/1
  Max Cold/1 -> Relational Operator11/1, Relational Operator5/1, Sum/1
  Relational Operator1/1 -> Logical Operator/2  "Bias Under 24.5mm  Increase Cold Up  Constant Force"
  Enable/1 -> Logical Operator8/1, Logical Operator5/2, Logical Operator4/2, Logical Operator1/1, Logical Operator/1
  Constant1/1 -> Relational Operator7/2, Relational Operator2/2
  Relational Operator2/1 -> Logical Operator1/2  "Bias Under 25.5mm Decrease Cold Up Constant Force"
  Bias/1 -> Relational Operator7/1, Sum/2, Relational Operator6/1, Relational Operator2/1, Relational Operator1/1
  Constant/1 -> Relational Operator6/2, Relational Operator1/2
  Relational Operator6/1 -> Logical Operator2/1
  Relational Operator7/1 -> Logical Operator2/2
  Logical Operator/1 -> Subsystem/1(In1)
  Subsystem/1(Out1) -> Increase Gain/1
  Logical Operator1/1 -> Subsystem1/1(In1)
  Subsystem1/1(Out1) -> Decrease Gain/1
  Logical Operator2/1 -> Logical Operator5/1, Logical Operator4/1, Logical Operator3/1  "24.5 <= Cold Bias <= 25.5"
  Sum2/1 -> Product1/1
  Logical Operator3/1 -> Data Type Conversion1/1
  Sum/1 -> Relational Operator4/1, Relational Operator10/1, Relational Operator9/1, Relational Operator8/1  "Amplitude"
  Constant2/1 -> Relational Operator9/2, Relational Operator4/2
  Logical Operator4/1 -> Subsystem2/1(In1)  "Amp<21 &&  Bias Balanced && Max Cold <TSL"
  Relational Operator4/1 -> Logical Operator4/3
  Relational Operator5/1 -> Logical Operator4/4
  Subsystem2/1(Out1) -> Increase Gain1/1
  Constant4/1 -> Relational Operator10/2, Relational Operator8/2
  Relational Operator8/1 -> Logical Operator5/3
  Logical Operator5/1 -> Subsystem3/1(In1)  "Amp > 22 && Bias Balanced"
  Subsystem3/1(Out1) -> Decrease Gain1/1
  Increase Gain1/1 -> Sum3/1
  Decrease Gain1/1 -> Sum3/2, Sum1/3
  Sum3/1 -> Product2/1
  Relational Operator9/1 -> Logical Operator6/1
  Relational Operator10/1 -> Logical Operator6/2
  Logical Operator6/1 -> Logical Operator7/1
  Logical Operator7/1 -> Product2/2
  Relational Operator11/1 -> Logical Operator8/2
  Logical Operator8/1 -> Subsystem4/1(In1)
  Subsystem4/1(Out1) -> Decrease Gain2/1
  Sum4/1 -> Sum1/2

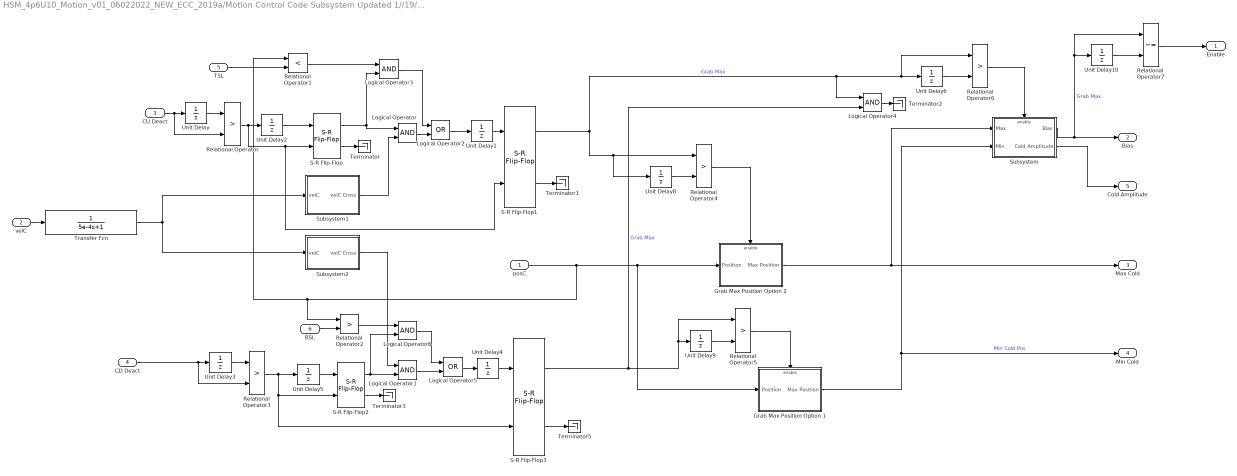
== system HSM_4p6U10_Motion_v01_06022022_NEW_ECC_2019a/Motion Control Code Subsystem Updated 1//19//21/Oscillation, Start Motion, 4 Phases Subsystem/Oscillations Subsystem Time pc No Cold Damping/Cold Resonance/Approximate Resonance Actuation/Calculate Cold Amp and Bias ==
  posC : Inport
  velC : Inport  Port=2
  CU Deact : Inport  Port=3
  CD Deact : Inport  Port=4
  TSL : Inport  Port=5
  BSL : Inport  Port=6
  Grab Max Position Option 1 : Subsystem
  Grab Max Position Option 2 : Subsystem
  Logical Operator{,1,3..4,6} (5 alike) : Logic  AllPortsSameDT=off  OutDataTypeStr=boolean
  Logical Operator2 : Logic  Operator=OR  AllPortsSameDT=off  OutDataTypeStr=boolean
  Logical Operator5 : Logic  Operator=OR  AllPortsSameDT=off  OutDataTypeStr=boolean
  Relational Operator{,2..6} (6 alike) : RelationalOperator  Operator=>  OutDataTypeStr=boolean  RndMeth=Simplest
  Relational Operator1 : RelationalOperator  Operator=<  OutDataTypeStr=boolean  RndMeth=Simplest
  Relational Operator7 : RelationalOperator  Operator=~=  OutDataTypeStr=boolean  RndMeth=Simplest
  S-R Flip-Flop{,1..3} (4 alike) : simulink_extras/Flip Flops/S-R Flip-Flop  initial_condition=0
  Subsystem : Subsystem
  Subsystem1 : Subsystem
  Subsystem2 : Subsystem
  Terminator{,1..3,5} (5 alike) : Terminator
  Transfer Fcn : TransferFcn  Denominator=[5e-4 1 ]
  Unit Delay{,1..6,8..10} (10 alike) : UnitDelay  SampleTime=-1  HasFrameUpgradeWarning=on
  Enable : Outport
  Bias : Outport  Port=2
  Max Cold : Outport  Port=3
  Min Cold : Outport  Port=4
  Cold Amplitude : Outport  Port=5
  wires:
  Subsystem/2(Cold Amplitude) -> Cold Amplitude/1
  S-R Flip-Flop3/1 -> Logical Operator4/2, Relational Operator5/1, Unit Delay9/1  "Grab Max"
  Unit Delay9/1 -> Relational Operator5/2
  Relational Operator5/1 -> Grab Max Position Option 1/Enable
  Relational Operator4/1 -> Grab Max Position Option 2/Enable
  Unit Delay8/1 -> Relational Operator4/2
  Transfer Fcn/1 -> Subsystem1/1(velC), Subsystem2/1(velC)
  Grab Max Position Option 2/1(Max Position) -> Max Cold/1, Subsystem/1(Max)
  BSL/1 -> Relational Operator2/2
  Relational Operator2/1 -> Logical Operator6/1
  Logical Operator6/1 -> Logical Operator5/1
  Logical Operator1/1 -> Logical Operator5/2
  Logical Operator3/1 -> Logical Operator2/1
  Relational Operator1/1 -> Logical Operator3/1
  TSL/1 -> Relational Operator1/2
  Logical Operator/1 -> Logical Operator2/2
  Unit Delay4/1 -> S-R Flip-Flop3/1
  Logical Operator5/1 -> Unit Delay4/1
  Subsystem2/1(velC Cross) -> Logical Operator1/1
  Unit Delay1/1 -> S-R Flip-Flop1/1
  Logical Operator2/1 -> Unit Delay1/1
  Subsystem1/1(velC Cross) -> Logical Operator/2
  Relational Operator6/1 -> Subsystem/Enable
  Unit Delay6/1 -> Relational Operator6/2
  Grab Max Position Option 1/1(Max Position) -> Subsystem/2(Min), Min Cold/1  "Min Cold Pos"
  posC/1 -> Relational Operator1/1, Relational Operator2/1, Grab Max Position Option 2/1(Position), Grab Max Position Option 1/1(Position)
  S-R Flip-Flop3/2 -> Terminator5/1
  S-R Flip-Flop2/2 -> Terminator3/1
  Relational Operator3/1 -> S-R Flip-Flop2/2, S-R Flip-Flop3/2, Unit Delay5/1
  CD Deact/1 -> Unit Delay3/1, Relational Operator3/2
  Unit Delay3/1 -> Relational Operator3/1
  S-R Flip-Flop2/1 -> Logical Operator1/2, Logical Operator6/2
  Unit Delay5/1 -> S-R Flip-Flop2/1
  S-R Flip-Flop1/1 -> Logical Operator4/1, Relational Operator6/1, Unit Delay6/1, Relational Operator4/1, Unit Delay8/1  "Grab Max"
  S-R Flip-Flop1/2 -> Terminator1/1
  Unit Delay2/1 -> S-R Flip-Flop/1
  S-R Flip-Flop/1 -> Logical Operator3/2, Logical Operator/1
  Unit Delay/1 -> Relational Operator/1
  CU Deact/1 -> Unit Delay/1, Relational Operator/2
  Relational Operator/1 -> Unit Delay2/1, S-R Flip-Flop/2, S-R Flip-Flop1/2
  S-R Flip-Flop/2 -> Terminator/1
  velC/1 -> Transfer Fcn/1
  Logical Operator4/1 -> Terminator2/1
  Subsystem/1(Bias) -> Unit Delay10/1, Relational Operator7/1, Bias/1  "Grab Max"
  Unit Delay10/1 -> Relational Operator7/2
  Relational Operator7/1 -> Enable/1

== system HSM_4p6U10_Motion_v01_06022022_NEW_ECC_2019a/Motion Control Code Subsystem Updated 1//19//21/Oscillation, Start Motion, 4 Phases Subsystem/Oscillations Subsystem Time pc No Cold Damping/Cold Resonance/Approximate Resonance Actuation/Subsystem1 ==
  Constant : Constant  Value=0.048
  Constant1 : Constant  Value=0.002
  Top Safety Limit : Outport
  Bottom Safety Limit : Outport  Port=2
  wires:
  Constant/1 -> Top Safety Limit/1  "Top Safety Limit"
  Constant1/1 -> Bottom Safety Limit/1  "Bottom Safety Limit"

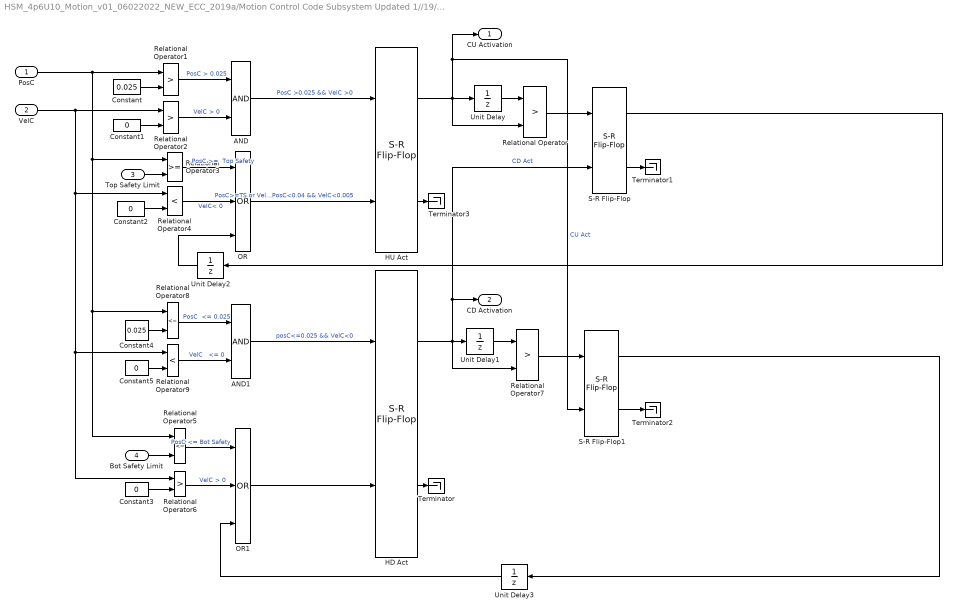
== system HSM_4p6U10_Motion_v01_06022022_NEW_ECC_2019a/Motion Control Code Subsystem Updated 1//19//21/Oscillation, Start Motion, 4 Phases Subsystem/Oscillations Subsystem Time pc No Cold Damping/Cold Resonance/Approximate Resonance Actuation/Subsystem2 ==
  PosC : Inport
  VelC : Inport  Port=2
  Top Safety Limit : Inport  Port=3
  Bot Safety Limit : Inport  Port=4
  AND : Logic  AllPortsSameDT=off  OutDataTypeStr=boolean
  AND1 : Logic  AllPortsSameDT=off  OutDataTypeStr=boolean
  Constant : Constant  Value=0.025
  Constant{1..3,5} (4 alike) : Constant  Value=0
  Constant4 : Constant  Value=0.025
  HD Act : simulink_extras/Flip Flops/S-R Flip-Flop  initial_condition=0
  HU Act : simulink_extras/Flip Flops/S-R Flip-Flop  initial_condition=0
  OR : Logic  Operator=OR  Inputs=3  AllPortsSameDT=off  OutDataTypeStr=boolean
  OR1 : Logic  Operator=OR  Inputs=3  AllPortsSameDT=off  OutDataTypeStr=boolean
  Relational Operator{,1..2,6..7} (5 alike) : RelationalOperator  Operator=>  OutDataTypeStr=boolean  RndMeth=Simplest
  Relational Operator3 : RelationalOperator  OutDataTypeStr=boolean  RndMeth=Simplest
  Relational Operator4 : RelationalOperator  Operator=<  OutDataTypeStr=boolean  RndMeth=Simplest
  Relational Operator5 : RelationalOperator  Operator=<=  OutDataTypeStr=boolean  RndMeth=Simplest
  Relational Operator8 : RelationalOperator  Operator=<=  OutDataTypeStr=boolean  RndMeth=Simplest
  Relational Operator9 : RelationalOperator  Operator=<  OutDataTypeStr=boolean  RndMeth=Simplest
  S-R Flip-Flop : simulink_extras/Flip Flops/S-R Flip-Flop  initial_condition=0
  S-R Flip-Flop1 : simulink_extras/Flip Flops/S-R Flip-Flop  initial_condition=0
  Terminator{,1..3} (4 alike) : Terminator
  Unit Delay{,1..3} (4 alike) : UnitDelay  SampleTime=-1  HasFrameUpgradeWarning=on
  CU Activation : Outport
  CD Activation : Outport  Port=2
  wires:
  Unit Delay3/1 -> OR1/3
  Unit Delay2/1 -> OR/3
  S-R Flip-Flop1/1 -> Unit Delay3/1
  S-R Flip-Flop1/2 -> Terminator2/1
  Relational Operator7/1 -> S-R Flip-Flop1/1
  Unit Delay1/1 -> Relational Operator7/1
  HD Act/1 -> S-R Flip-Flop/2, CD Activation/1, Relational Operator7/2, Unit Delay1/1  "CD Act"
  S-R Flip-Flop/1 -> Unit Delay2/1
  S-R Flip-Flop/2 -> Terminator1/1
  Relational Operator/1 -> S-R Flip-Flop/1
  Unit Delay/1 -> Relational Operator/1
  HU Act/1 -> Unit Delay/1, S-R Flip-Flop1/2, CU Activation/1, Relational Operator/2  "CU Act"
  Relational Operator8/1 -> AND1/1  "PosC  <= 0.025"
  Constant4/1 -> Relational Operator8/2
  VelC/1 -> Relational Operator2/1, Relational Operator4/1, Relational Operator9/1, Relational Operator6/1
  Constant5/1 -> Relational Operator9/2
  Relational Operator9/1 -> AND1/2  "VelC   <= 0"
  AND1/1 -> HD Act/1  "posC<=0.025 && VelC<0"
  PosC/1 -> Relational Operator1/1, Relational Operator3/1, Relational Operator8/1, Relational Operator5/1
  AND/1 -> HU Act/1  "PosC >0.025 && VelC >0"
  Bot Safety Limit/1 -> Relational Operator5/2
  Relational Operator5/1 -> OR1/1  "PosC <= Bot Safety"
  Constant3/1 -> Relational Operator6/2
  Relational Operator6/1 -> OR1/2  "VelC > 0"
  OR1/1 -> HD Act/2
  OR/1 -> HU Act/2  "PosC>=TS or VelC<0 or  PosC<0.04 && VelC<0.005"
  Relational Operator4/1 -> OR/2  "VelC< 0"
  Constant2/1 -> Relational Operator4/2
  Relational Operator3/1 -> OR/1  "PosC >=  Top Safety"
  Top Safety Limit/1 -> Relational Operator3/2
  Constant1/1 -> Relational Operator2/2
  Relational Operator2/1 -> AND/2  "VelC > 0"
  Relational Operator1/1 -> AND/1  "PosC > 0.025"
  Constant/1 -> Relational Operator1/2
  HD Act/2 -> Terminator/1
  HU Act/2 -> Terminator3/1

== system HSM_4p6U10_Motion_v01_06022022_NEW_ECC_2019a/Motion Control Code Subsystem Updated 1//19//21/Oscillation, Start Motion, 4 Phases Subsystem/Oscillations Subsystem Time pc No Cold Damping/Cold Resonance/Cold Down Control/Unity Gain Scaling ==
  u : Inport
  x : Inport  Port=2
  Constant6 : Constant  Value=K2m
  Gain1 : Gain  Gain=-1/K1m
  IBC^2 Saturation : Saturate  UpperLimit=1600  LowerLimit=0
  Math Function4 : Math  Operator=square  SaturateOnIntegerOverflow=on
  Product1 : Product
  Sqrt : Sqrt  SaturateOnIntegerOverflow=on
  Sum3 : Sum
  i : Outport
  wires:
  IBC^2 Saturation/1 -> Sqrt/1
  Sqrt/1 -> i/1
  Product1/1 -> IBC^2 Saturation/1
  Gain1/1 -> Product1/1
  x/1 -> Sum3/2
  Math Function4/1 -> Product1/2
  Constant6/1 -> Sum3/1
  Sum3/1 -> Math Function4/1
  u/1 -> Gain1/1

== system HSM_4p6U10_Motion_v01_06022022_NEW_ECC_2019a/Motion Control Code Subsystem Updated 1//19//21/Oscillation, Start Motion, 4 Phases Subsystem/Oscillations Subsystem Time pc No Cold Damping/Cold Resonance/Cold Up Control/Acceleration to Current ==
  U : Inport
  X : Inport  Port=2
  Constant6 : Constant  Value=K2m+0.05
  Gain1 : Gain  Gain=1/K1m
  IRC^2 Saturation : Saturate  UpperLimit=1600  LowerLimit=0
  Math Function4 : Math  Operator=square  SaturateOnIntegerOverflow=on
  Product1 : Product
  Sqrt : Sqrt  SaturateOnIntegerOverflow=on
  Sum3 : Sum  Inputs=+-
  I : Outport
  wires:
  U/1 -> Gain1/1
  IRC^2 Saturation/1 -> Sqrt/1
  Sum3/1 -> Math Function4/1
  Constant6/1 -> Sum3/1
  Math Function4/1 -> Product1/2
  X/1 -> Sum3/2
  Gain1/1 -> Product1/1
  Product1/1 -> IRC^2 Saturation/1
  Sqrt/1 -> I/1
